simulink model "pump_soft_sensor"  (R2019b)
settings: Solver=FixedStepAuto  StartTime=0.0  StopTime=10.0  RelTol=1e-3
libraries: fl_lib x6, nesl_utility x5, sh_lib x4
settings Model: Creator=z0047h2k  LastModifiedBy=z0047h2k
settings HardwareCC: ProdBitPerLong=64  ProdLongLongMode=on  ProdHWDeviceType=Intel->x86-64 (Linux 64)
settings RTWCC: PackageGeneratedCodeAndArtifacts=on  PackageName=pump_soft_sensor  Toolchain=Microsoft Visual C++ 2019 v16.0 | nmake (64-bit Windows)  BuildConfiguration=Faster Runs  TargetLang=C++
settings GRTTargetCC: TargetLangStandard=C++03 (ISO)  MatFileLogging=off  MultiInstanceERTCode=on  CodeInterfacePackaging=C++ class  RTWCAPISignals=on  RTWCAPIParams=on  RTWCAPIStates=on  RTWCAPIRootIO=on

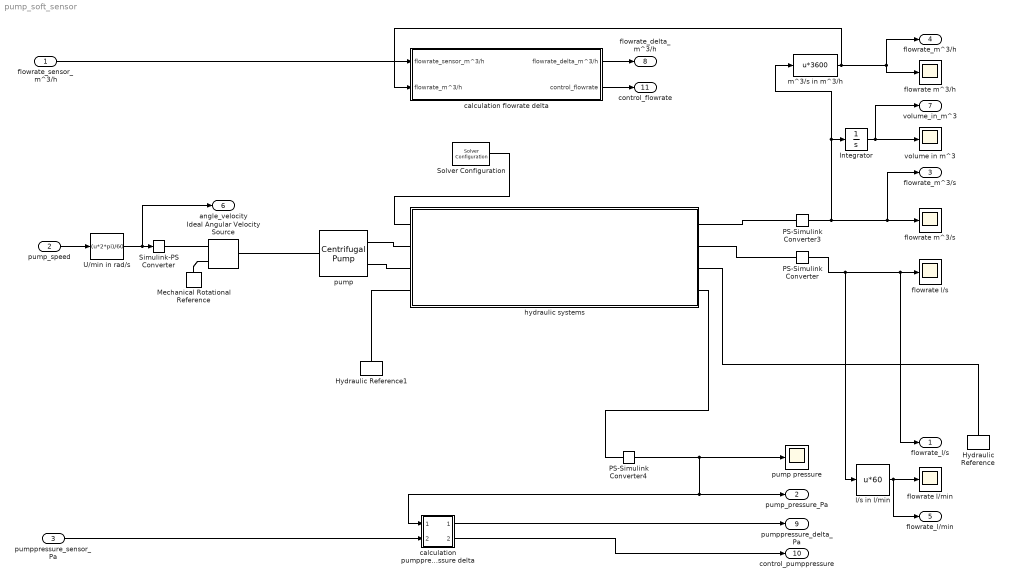
== system pump_soft_sensor ==
  flowrate_sensor_m^3/h : Inport
  pump_speed : Inport  Port=2
  pumppressure_sensor_Pa : Inport  Port=3
  Hydraulic Reference : fl_lib/Hydraulic/Hydraulic Elements/Hydraulic Reference
      settings: SourceProductName=Simscape
  Hydraulic Reference1 : fl_lib/Hydraulic/Hydraulic Elements/Hydraulic Reference
      settings: SourceProductName=Simscape
  Ideal Angular Velocity Source : fl_lib/Mechanical/Mechanical Sources/Ideal Angular Velocity Source
  Integrator : Integrator
  Mechanical Rotational Reference : fl_lib/Mechanical/Rotational Elements/Mechanical Rotational Reference
  PS-Simulink Converter : nesl_utility/PS-Simulink Converter  PhysicalDomain=network_engine_domain  SubClassName=ps_output  LeftPortType=input  RightPortType=output  PseudoPeriodic=off  Frequencies=[]  Unit=inherit  AffineConversion=off
  PS-Simulink Converter3 : nesl_utility/PS-Simulink Converter  PhysicalDomain=network_engine_domain  SubClassName=ps_output  LeftPortType=input  RightPortType=output  PseudoPeriodic=off  Frequencies=[]  Unit=inherit  AffineConversion=off
  PS-Simulink Converter4 : nesl_utility/PS-Simulink Converter  PhysicalDomain=network_engine_domain  SubClassName=ps_output  LeftPortType=input  RightPortType=output  PseudoPeriodic=off  Frequencies=[]  Unit=inherit  AffineConversion=off
  Simulink-PS Converter : nesl_utility/Simulink-PS Converter  PhysicalDomain=network_engine_domain  SubClassName=ps_input  LeftPortType=input  RightPortType=output  PseudoPeriodic=off  Frequencies=[]  NoiseDistribution=none  NoiseParameters=[]  Unit=1  AffineConversion=off  FilteringAndDerivatives=provide  SimscapeFilterOrder=1  InputFilterTimeConstant=0.001  UdotUserProvided=0
  Solver Configuration : nesl_utility/Solver Configuration  PhysicalDomain=network_engine_domain  SubClassName=solver  LeftPortType=input  RightPortType=generic  Tones=[]  Harmonics=[]  SimulateNoise=off  Profile=off  UseLocalSampling=off  EnableSwitchedLinearOptims=on  FrequencyDomain=off  UseCCode=off  RelTol=0.001  AbsTol=1e-06  MinStep=1e-09  ToWorkspace=off  RevertToSquareIcSolve=off  NumHomotopyIterations=100  PhasorMode=off  PhasorModeNumHarmonics=1  DoDC=off  ResidualTolerance=1e-09  UseLocalSolver=on  LocalSolverChoice=NE_PARTITIONING_ADVANCER  LocalSolverSampleTime=0.001  DoFixedCost=on  MaxNonlinIter=3  MaxModeIter=2  LinearAlgebra=auto  EquationFormulation=NE_TIME_EF  DelaysMemoryBudget=1024  AutomaticFiltering=on  FilteringTimeConstant=0.001  PartitionStorageMethod=AS_NEEDED  PartitionMemoryBudget=1024  PartitionMethod=ROBUST
  U/min in rad/s : Fcn  Expr=(u*2*pi)/60
  calculation flowrate delta : Subsystem
  calculation pumppressure delta : Subsystem
  flowrate l/min : Scope
  flowrate l/s : Scope
  flowrate m^3/h : Scope
  flowrate m^3/s : Scope
  hydraulic systems : Subsystem
  l/s in l/min : Fcn  Expr=u*60
  m^3/s in m^3/h : Fcn  Expr=u*3600
  pump : sh_lib/Pumps and Motors/Centrifugal Pump  mdl_type=2  c_1=First_approximation_coefficient Pa/(kg/m^3)  c_2=Second_approximation_coefficient Pa*s/kg  c_3=Theird_approximation_coefficient Pa*s^2/(kg*m^3)  c_4=Fourth_approximation_coefficient Pa*s^2/(kg*m^3)  c_f=Correction_factor  design_del=Pump_design_delivery lpm  ref_velocity=Reference_angular_velocity rpm  ref_density=Reference_density kg/m^3  leak_resistance=Leak_resistance Pa/(m^3/s)  T_const=Drive_shaft_torque N*m  trq_press_coeff=Torque_pressure_coefficient N*m/Pa  pump_del_1D=pump_delivery_vector_pressure_differential lpm  press_diff_1D=pump_pressure_differential_vector bar  pump_del_power_1D=pump_delivery_vector_brake_power lpm  power_1D=pump_brake_power_vector kW  pump_vel_2D=[3200, 3300, 3400, 3500] rpm  pump_del_2D=[0, 50, 100, 150, 200, 250, 300, 350] lpm  press_diff_2D=[8.3, 8.8, 9.3, 9.9; 7.8, 8.3, 8.8, 9.4; 7.2, 7.6, 8.2, 8.7; 6.5, 7, 7.5, 8; 5.6, 6.1, 6.6, 7.1; 4.7, 5.2, 5.7, 6.2; 3.4, 4, 4.4, 4.9; 2.3, 2.7, 3.4, 3.6] bar  pump_del_power_2D=[0, 50, 100, 150, 200, 250, 300, 350] lpm  power_2D=[1223, 1341, 1467, 1600; 1414, 1551, 1696, 1850; 1636, 1794, 1962, 2140; 1941, 2129, 2326, 2540; 2224, 2439, 2660, 2910; 2453, 2691, 2947, 3210; 2757, 3024, 3307, 3608; 2945, 3230, 3533, 3854] W  omega_threshold=Angular_speed_treshold_for_flow_reversal rad/s  interp_method=1  extrap_method=1
      settings: SourceProductName=Simscape Fluids  SourceProductBaseCode=SH  LogSimulationData=on  InternalSimscapePortConfiguration="{\"Bottom\":[],\"Left\":[{\"id\":\"S\",\"label\":\"S\",\"type\":\"foundation.mechanical.rotational.rotational\"}],\"Right\":[{\"id\":\"P\",\"label\":\"P\",\"type\":\"foundation.hydraulic.hydraulic\"},{\"id\":\"T\",\"label\":\"T\",\"type\":\"foundation.hydraulic.hydraulic\"}],\"Top\":[]}"
  pump pressure : Scope
  volume in m^3 : Scope
  flowrate_l/s : Outport
  pump_pressure_Pa : Outport  Port=2
  flowrate_m^3/s : Outport  Port=3
  flowrate_m^3/h : Outport  Port=4
  flowrate_l/min : Outport  Port=5
  angle_velocity : Outport  Port=6
  volume_in_m^3 : Outport  Port=7
  flowrate_delta_m^3/h : Outport  Port=8
  pumppressure_delta_Pa : Outport  Port=9
  control_pumppressure : Outport  Port=10
  control_flowrate : Outport  Port=11
  wires:
  l/s in l/min/1 -> flowrate_l/min/1, flowrate l/min/1
  calculation pumppressure delta/2(control_pumppressure) -> control_pumppressure/1
  calculation pumppressure delta/1(pumppressure_delta_Pa) -> pumppressure_delta_Pa/1
  PS-Simulink Converter4/1 -> pump pressure/1, calculation pumppressure delta/1(pump_pressure_Pa), pump_pressure_Pa/1
  U/min in rad/s/1 -> angle_velocity/1, Simulink-PS Converter/1
  calculation flowrate delta/1(flowrate_delta_m^3/h) -> flowrate_delta_m^3/h/1
  pumppressure_sensor_Pa/1 -> calculation pumppressure delta/2(pumppressure_Sensor_Pa)
  calculation flowrate delta/2(control_flowrate) -> control_flowrate/1
  flowrate_sensor_m^3/h/1 -> calculation flowrate delta/1(flowrate_sensor_m^3/h)
  m^3/s in m^3/h/1 -> flowrate_m^3/h/1, flowrate m^3/h/1, calculation flowrate delta/2(flowrate_m^3/h)
  PS-Simulink Converter/1 -> flowrate l/s/1, flowrate_l/s/1, l/s in l/min/1
  Integrator/1 -> volume_in_m^3/1, volume in m^3/1
  PS-Simulink Converter3/1 -> m^3/s in m^3/h/1, Integrator/1, flowrate_m^3/s/1, flowrate m^3/s/1
  pump_speed/1 -> U/min in rad/s/1
  connections:
  hydraulic systems/RConn1 -- PS-Simulink Converter3/LConn1
  Hydraulic Reference/LConn1 -- hydraulic systems/RConn3
  hydraulic systems/RConn2 -- PS-Simulink Converter/LConn1
  Ideal Angular Velocity Source/RConn2 -- Mechanical Rotational Reference/LConn1
  pump/RConn1 -- hydraulic systems/LConn2
  PS-Simulink Converter4/LConn1 -- hydraulic systems/RConn4
  hydraulic systems/LConn4 -- Hydraulic Reference1/LConn1
  Simulink-PS Converter/RConn1 -- Ideal Angular Velocity Source/RConn1
  Solver Configuration/RConn1 -- hydraulic systems/LConn1
  pump/LConn1 -- Ideal Angular Velocity Source/LConn1
  hydraulic systems/LConn3 -- pump/RConn2

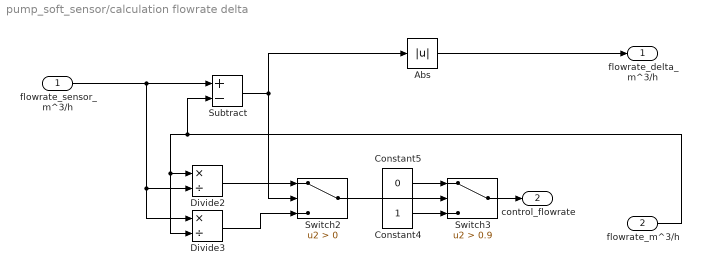
== system pump_soft_sensor/calculation flowrate delta ==
  flowrate_sensor_m^3/h : Inport
  flowrate_m^3/h : Inport  Port=2
  Abs : Abs
  Constant4 : Constant
  Constant5 : Constant  Value=0
  Divide2 : Product  Inputs=*/
  Divide3 : Product  Inputs=*/
  Subtract : Sum  Inputs=+-
  Switch2 : Switch  Criteria=u2 > Threshold
  Switch3 : Switch  Criteria=u2 > Threshold  Threshold=0.9
  flowrate_delta_m^3/h : Outport
  control_flowrate : Outport  Port=2
  wires:
  Divide3/1 -> Switch2/3
  Constant5/1 -> Switch3/1
  flowrate_m^3/h/1 -> Divide3/2, Divide2/1, Subtract/2
  flowrate_sensor_m^3/h/1 -> Divide3/1, Divide2/2, Subtract/1
  Subtract/1 -> Abs/1, Switch2/2
  Switch3/1 -> control_flowrate/1
  Switch2/1 -> Switch3/2
  Divide2/1 -> Switch2/1
  Constant4/1 -> Switch3/3
  Abs/1 -> flowrate_delta_m^3/h/1

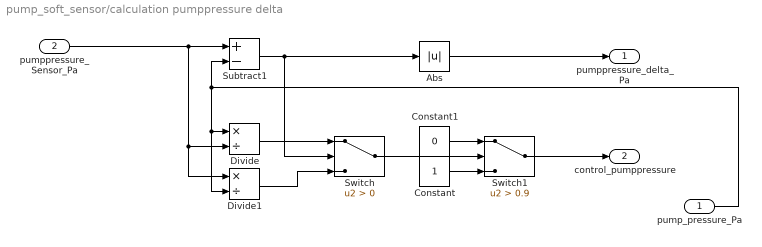
== system pump_soft_sensor/calculation pumppressure delta ==
  pump_pressure_Pa : Inport
  pumppressure_Sensor_Pa : Inport  Port=2
  Abs : Abs
  Constant : Constant
  Constant1 : Constant  Value=0
  Divide : Product  Inputs=*/
  Divide1 : Product  Inputs=*/
  Subtract1 : Sum  Inputs=+-
  Switch : Switch  Criteria=u2 > Threshold
  Switch1 : Switch  Criteria=u2 > Threshold  Threshold=0.9
  pumppressure_delta_Pa : Outport
  control_pumppressure : Outport  Port=2
  wires:
  Subtract1/1 -> Abs/1, Switch/2
  Divide/1 -> Switch/1
  pumppressure_Sensor_Pa/1 -> Divide1/1, Divide/2, Subtract1/1
  Switch/1 -> Switch1/2
  pump_pressure_Pa/1 -> Subtract1/2, Divide1/2, Divide/1
  Constant1/1 -> Switch1/1
  Constant/1 -> Switch1/3
  Divide1/1 -> Switch/3
  Switch1/1 -> control_pumppressure/1
  Abs/1 -> pumppressure_delta_Pa/1

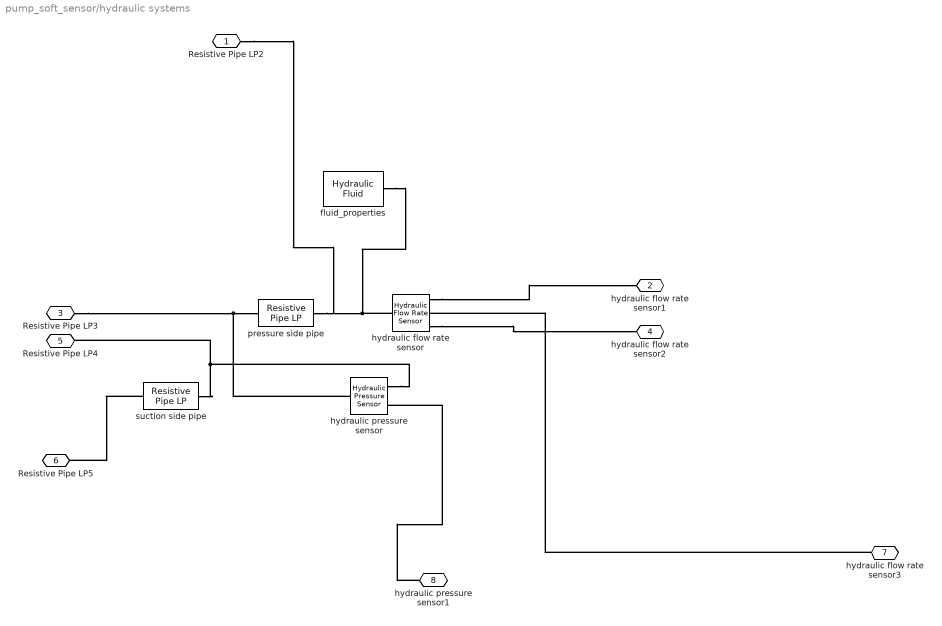
== system pump_soft_sensor/hydraulic systems ==
  fluid_properties : sh_lib/Hydraulic Utilities/Hydraulic Fluid  DataSource=1  SelFluid=24  SysTemp=20  TrapAir=0.005  ViscDerFactor=1  range_error=2
      settings: SourceProductName=Simscape Fluids
  hydraulic flow rate sensor : fl_lib/Hydraulic/Hydraulic Sensors/Hydraulic Flow Rate Sensor
      settings: SourceProductName=Simscape  LogSimulationData=on
  hydraulic pressure sensor : fl_lib/Hydraulic/Hydraulic Sensors/Hydraulic Pressure Sensor
      settings: SourceProductName=Simscape
  pressure side pipe : sh_lib/Low-Pressure Blocks/Resistive Pipe LP  cs_type=1  d_in=pressure_pipe_internal_diameter m  area=1e-4 m^2  D_h=1.12e-2 m  s_factor=64  length=pressure_pipe_length m  length_ad=1 m  roughness=15e-6 m  Re_lam=2000  Re_turb=4000  elevation_A=pressure_pipe_inlet_heigth m  elevation_B=pressure_pipe_outlet_heigth m  g=9.80665 m/s^2  pressure_drop_specify=off  pressure_drop_priority=None  pressure_drop=0 Pa  pressure_drop_nominal_specify=off  pressure_drop_nominal_unit=Pa  pressure_drop_nominal_value=1  flow_rate_specify=off  flow_rate_priority=None  flow_rate=0 m^3/s  flow_rate_nominal_specify=off  flow_rate_nominal_unit=m^3/s  flow_rate_nominal_value=1
      settings: SourceProductName=Simscape Fluids  SourceProductBaseCode=SH  InternalSimscapePortConfiguration="{\"Bottom\":[],\"Left\":[{\"id\":\"A\",\"label\":\"A\",\"type\":\"foundation.hydraulic.hydraulic\"}],\"Right\":[{\"id\":\"B\",\"label\":\"B\",\"type\":\"foundation.hydraulic.hydraulic\"}],\"Top\":[]}"
  suction side pipe : sh_lib/Low-Pressure Blocks/Resistive Pipe LP  cs_type=1  d_in=suction_pipe_internal_diameter m  area=1e-4 m^2  D_h=1.12e-2 m  s_factor=64  length=suction_pipe_length m  length_ad=1 m  roughness=15e-6 m  Re_lam=2000  Re_turb=4000  elevation_A=suction_pipe_inlet_heigth m  elevation_B=suction_pipe_outlet_heigth m  g=9.80665 m/s^2  pressure_drop_specify=off  pressure_drop_priority=None  pressure_drop=0 Pa  pressure_drop_nominal_specify=off  pressure_drop_nominal_unit=Pa  pressure_drop_nominal_value=1  flow_rate_specify=off  flow_rate_priority=None  flow_rate=0 m^3/s  flow_rate_nominal_specify=off  flow_rate_nominal_unit=m^3/s  flow_rate_nominal_value=1
      settings: SourceProductName=Simscape Fluids  SourceProductBaseCode=SH  InternalSimscapePortConfiguration="{\"Bottom\":[],\"Left\":[{\"id\":\"A\",\"label\":\"A\",\"type\":\"foundation.hydraulic.hydraulic\"}],\"Right\":[{\"id\":\"B\",\"label\":\"B\",\"type\":\"foundation.hydraulic.hydraulic\"}],\"Top\":[]}"
  Resistive Pipe LP2 : PMIOPort  Side=Left
  hydraulic flow rate sensor1 : PMIOPort  Port=2  Side=Right
  Resistive Pipe LP3 : PMIOPort  Port=3  Side=Left
  hydraulic flow rate sensor2 : PMIOPort  Port=4  Side=Right
  Resistive Pipe LP4 : PMIOPort  Port=5  Side=Left
  Resistive Pipe LP5 : PMIOPort  Port=6  Side=Left
  hydraulic flow rate sensor3 : PMIOPort  Port=7  Side=Right
  hydraulic pressure sensor1 : PMIOPort  Port=8  Side=Right
  connections:
  hydraulic pressure sensor/RConn1 -- Resistive Pipe LP4/RConn1 -- suction side pipe/RConn1
  hydraulic flow rate sensor3/RConn1 -- hydraulic flow rate sensor/RConn2
  hydraulic flow rate sensor/LConn1 -- fluid_properties/RConn1 -- Resistive Pipe LP2/RConn1 -- pressure side pipe/RConn1
  hydraulic pressure sensor/LConn1 -- Resistive Pipe LP3/RConn1 -- pressure side pipe/LConn1
  suction side pipe/LConn1 -- Resistive Pipe LP5/RConn1
  hydraulic pressure sensor1/RConn1 -- hydraulic pressure sensor/RConn2
  hydraulic flow rate sensor/RConn3 -- hydraulic flow rate sensor2/RConn1
  hydraulic flow rate sensor/RConn1 -- hydraulic flow rate sensor1/RConn1
